simulink model "kf_discrete_time_2017"  (R2017b)
settings: Solver=FixedStepAuto  StartTime=0.0  StopTime=15  FixedStep=1e-3  RelTol=1e-3
values from neighbouring files (symbols this model uses):
  Ts = 0.1    [KinematicBicycleModel.m]    (also in LeftLaneChangeSinusoidalMotionModel.m; LinearizedBicycleModel.m; SimplifiedKinematicBicycleModel.m; amm_rel_test.m)
  vx = X(2)    [cv_model_fun.m]    (also in initialization.m = 10)
  vy = X(4)    [cv_model_fun.m]    (also in initialization.m = 0)
  x = X(1)    [KinematicBicycleModel.m]    (also in SimplifiedKinematicBicycleModel.m; behavior_model.m = 0:0.01:20; cca_model_fun.m; ctra_model_fun.m)
  y = X(2)    [KinematicBicycleModel.m]    (also in SimplifiedKinematicBicycleModel.m; behavior_model.m = [distances velocities]; cca_model_fun.m; ctra_model_fun.m)
undefined symbols (not defined in the file or in its folder): Discrete, Time
libraries: ctrlSharedLib x1, dspadpt3 x1, simulink x1
settings Model: Creator=jasprit  LastModifiedBy=jasprit

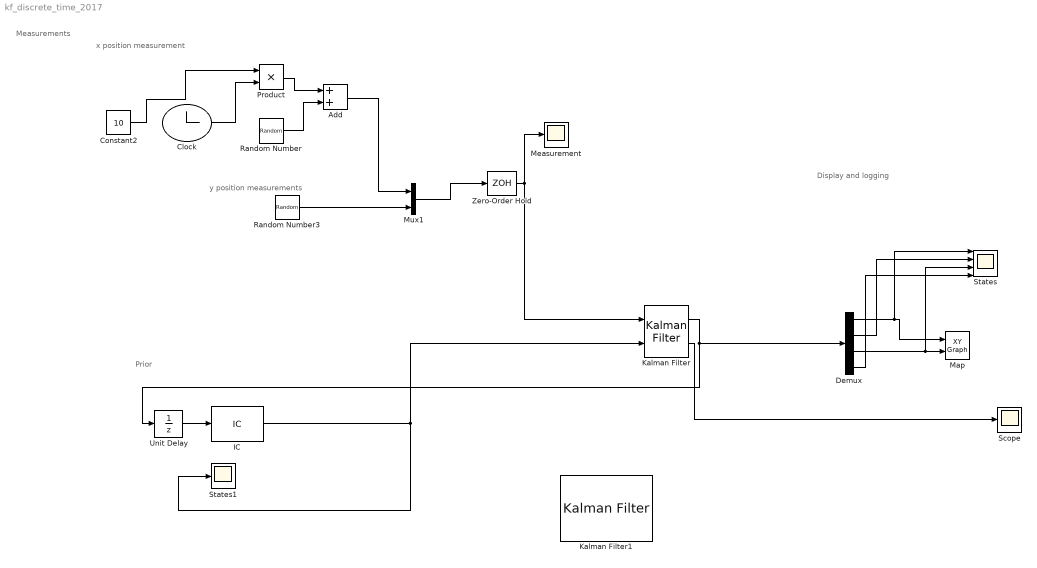
== system kf_discrete_time_2017 ==
  note: y position measurements
  note: x position measurement
  note: Display and logging
  note: Prior
  note: Measurements
  Add : Sum
  Clock : Clock
  Constant2 : Constant  Value=10
  Demux : Demux
  IC : InitialCondition  Value=[x vx y vy]'
  Kalman Filter : ctrlSharedLib/Kalman Filter  TimeDomain=Discrete-Time  UseCurrentEstimator=on  ModelSource=Individual A, B, C, D matrices  ModelSourceVariable=ss(0.95,1,1,0,1)  A=[1 Ts 0 0; 0 1 0 0; 0 0 1 Ts; 0 0 0 1]  B=[1 0; 0 1]  C=[1 0 0 0; 0 0 1 0]  D=[0 0; 0 0]  NumberOfStates=1  NumberOfInputs=1  NumberOfOutputs=1  InitialEstimateSource=Input port  X0=[0 0 20 0]  P0=10  UseK=off  UseGH=off  NumberOfProcessNoiseInputs=1  G=1  TimeInvariantG=on  H=0  TimeInvariantH=on  Q=[0.5 5 0.5 5]'  TimeInvariantQ=on  R=[0.2 0; 0 0.2]  TimeInvariantR=on  N=0  TimeInvariantN=on  AddInputPort=off  AddEnablePort=off  OutputEstimatedY=off  OutputP=on  Ts=Ts
      settings: SourceProductBaseCode=CT
  Kalman Filter1 : dspadpt3/Kalman Filter  num_targets=10  sourceEnable=Specify via input port <Enable>  isReset=on  X=zeros([6, 1])  P=10*eye(6)  A=[1 0 1 0 0 0;0 1 0 1 0 0; 0 0 1 0 0 0; 0 0 0 1 0 0; 0 0 0 0 1 0; 0 0 0 0 0 1]  sourceMeasure=Specify via Dialog  H=[1 0 0 0 0 0; 0 1 0 0 0 0; 0 0 0 0 1 0; 0 0 0 0 0 1]  Q=0.05*eye(6)  R=eye(4)  isOutputEstMeasure=on  isOutputEstState=off  isOutputEstError=off  isOutputPrdMeasure=off  isOutputPrdState=off  isOutputPrdError=off
      settings: SourceProductName=DSP System Toolbox  SourceProductBaseCode=DS
  Map : simulink/Sinks/XY Graph  xmin=-1  xmax=200  ymin=-20  ymax=20  st=-1
  "Measurement " : Scope
  Mux1 : Mux  Inputs=2
  Product : Product
  Random Number : RandomNumber  Variance=0.1  SampleTime=Ts
  Random Number3 : RandomNumber  Variance=0.2  SampleTime=Ts
  Scope : Scope
  States : Scope  NumInputPorts=4
  States1 : Scope
  Unit Delay : UnitDelay  SampleTime=-1
  Zero-Order Hold : ZeroOrderHold  SampleTime=Ts
  wires:
  Constant2/1 -> Product/1
  Kalman Filter/1 -> Unit Delay/1, Demux/1
  Demux/1 -> States/1, Map/1
  Clock/1 -> Product/2
  Product/1 -> Add/1
  Random Number/1 -> Add/2
  Add/1 -> Mux1/1
  Kalman Filter/2 -> Scope/1
  Demux/2 -> States/2
  Mux1/1 -> Zero-Order Hold/1
  Random Number3/1 -> Mux1/2
  Demux/3 -> Map/2, States/3
  Demux/4 -> States/4
  IC/1 -> States1/1, Kalman Filter/2
  Zero-Order Hold/1 -> Kalman Filter/1, "Measurement "/1
  Unit Delay/1 -> IC/1
